simulink model "qftdm2_sim"  (Simulink 5.0)
settings: Solver=ode45  StartTime=0.0  StopTime=5  RelTol=1e-3
values from neighbouring files (symbols this model uses):
  k = size(q)    [chap8_4armplot.m]    (also in chap8_5ctrl.m = 30; chap8_6ctrl.m = 2; qft_int.m = 1; qftdm1_int.m = 379)
  p1 = 123.5+213.9i    [qftdm1_int.m]    (also in qftdm2_int.m = 42.81)
  p2 = P(1,2)    [chap8_1ctrl.m]    (also in chap8_2ctrl.m; qftdm1_int.m = 123.5-213.9i; qftdm2_int.m = 743+669.3i)
  p3 = P(2,2)    [chap8_1ctrl.m]    (also in chap8_2ctrl.m; qftdm2_int.m = 743-669.3i)
  pf1 = 2.8+2.857i    [qftdm2_int.m]
  pf2 = 2.8-2.857i    [qftdm2_int.m]
  z1 = 42    [qftdm1_int.m]    (also in qftdm2_int.m = 1.1)
  z2 = 113.8    [qftdm2_int.m]
libraries: simulink x1
settings Model: LastModifiedBy=Administrator  ExtModeTrigMode=oneshot  ExtModeArmWhenConnect=off  LimitDataPoints=off  BooleanDataType=off

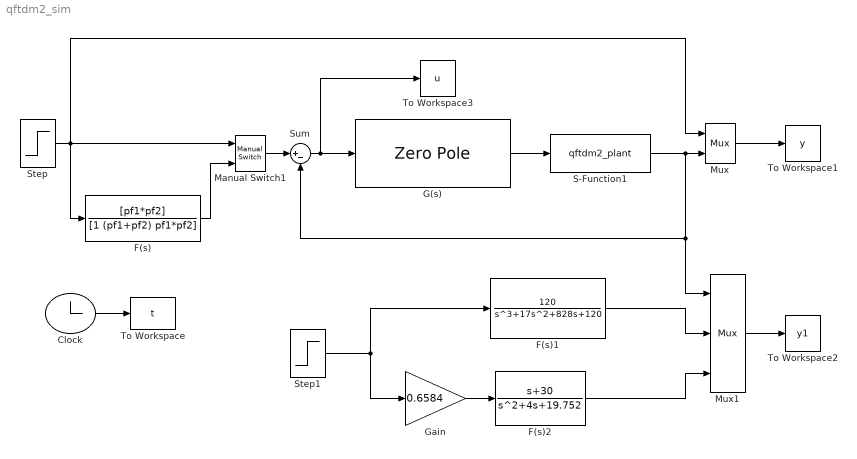
== system qftdm2_sim ==
  Clock : Clock
  F(s) : TransferFcn  Numerator=[pf1*pf2]  Denominator=[1 (pf1+pf2) pf1*pf2]
  F(s)1 : TransferFcn  Numerator=[120]  Denominator=[1 17 828 120]
  F(s)2 : TransferFcn  Numerator=[1 30]  Denominator=[1 4 19.752]
  G(s) : ZeroPole  Zeros=[-z1 -z2]  Poles=[-p1 -p2 -p3]  Gain=[k*p1*p2*p3/(z1*z2)]
  Gain : Gain  Gain=0.6584  SaturateOnIntegerOverflow=on
  Manual Switch1 : simulink/Signal Routing/Manual Switch  sw=0  action=0
  Mux : Mux  Inputs=2
  Mux1 : Mux  Inputs=3
  S-Function1 : S-Function  FunctionName=qftdm2_plant
  Step : Step  Time=0  SampleTime=0
  Step1 : Step  Time=0  SampleTime=0
  Sum : Sum  Inputs=|+-  SaturateOnIntegerOverflow=on  InputSameDT=on
  To Workspace : ToWorkspace  VariableName=t  SampleTime=-1  SaveFormat=Array
  To Workspace1 : ToWorkspace  VariableName=y  SampleTime=-1  SaveFormat=Array
  To Workspace2 : ToWorkspace  VariableName=y1  SampleTime=-1  SaveFormat=Array
  To Workspace3 : ToWorkspace  VariableName=u  SampleTime=-1  SaveFormat=Array
  wires:
  S-Function1/1 -> Mux/2, Sum/2, Mux1/1
  Mux/1 -> To Workspace1/1
  Sum/1 -> G(s)/1, To Workspace3/1
  Manual Switch1/1 -> Sum/1
  F(s)/1 -> Manual Switch1/2
  Step/1 -> Mux/1, F(s)/1, Manual Switch1/1
  G(s)/1 -> S-Function1/1
  Clock/1 -> To Workspace/1
  Gain/1 -> F(s)2/1
  Step1/1 -> Gain/1, F(s)1/1
  Mux1/1 -> To Workspace2/1
  F(s)1/1 -> Mux1/2
  F(s)2/1 -> Mux1/3
